simulink model "pm_motor"  (R2022b)
settings: Solver=VariableStepAuto  StartTime=0.0  StopTime=10.0  RelTol=1e-3
values from neighbouring files (symbols this model uses):
  fe = Phif    (= 2.3036)    [pm_params.m]
  J = 0.013    [IM_System_1.m]    (also in IM_System_2.m; IM_System_3.m; IM_System_noPU_4p2p2kw.m; IM_System_noPU_4p2p2kw_1.m)
  Ld = 0.006    [SPM_System_noPU_3p7kw_PI.m]    (also in pm_params.m = 0.8643)
  Lq = 0.0149    [SPM_System_noPU_3p7kw_PI.m]    (also in pm_params.m = 0.8643)
  Rs = 2.5/3    (= 0.833333333333)    [IM_System_1.m]    (also in IM_System_2.m; IM_System_3.m; IM_System_noPU_4p2p2kw.m; IM_System_noPU_4p2p2kw_1.m)
settings Model: Creator=jack  LastModifiedBy=jack

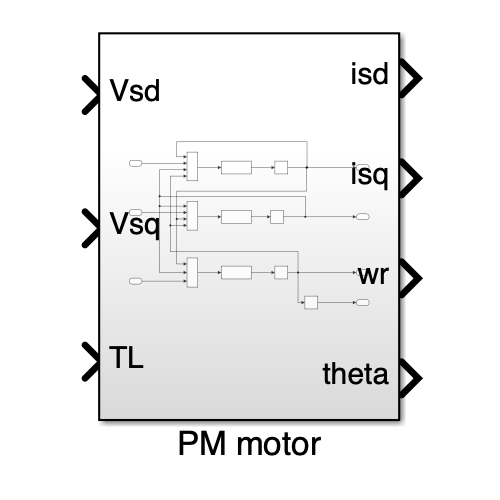
[thumbnail: Simulink's stored preview of the top-level diagram]
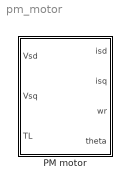
== system pm_motor ==
  PM motor : Subsystem

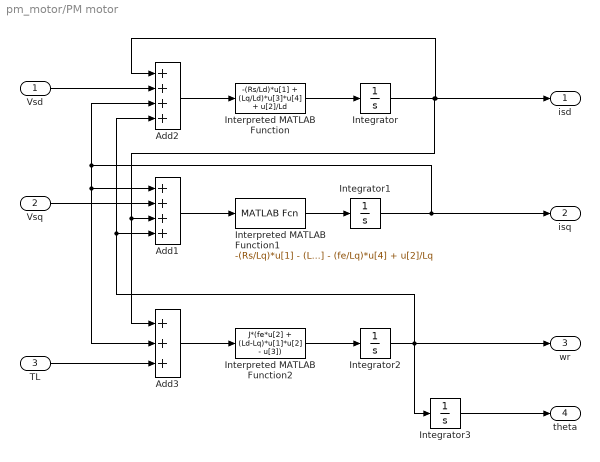
== system pm_motor/PM motor ==
  Vsd : Inport
  Vsq : Inport  Port=2
  TL : Inport  Port=3
  Add1 : Sum  Inputs=++++
  Add2 : Sum  Inputs=++++
  Add3 : Sum  Inputs=+++
  Integrator{,1..3} (4 alike) : Integrator
  Interpreted MATLAB Function : MATLABFcn  MATLABFcn=-(Rs/Ld)*u[1] + (Lq/Ld)*u[3]*u[4] + u[2]/Ld
  Interpreted MATLAB Function1 : MATLABFcn  MATLABFcn=-(Rs/Lq)*u[1] - (Ld/Lq)*u[3]*u[4] - (fe/Lq)*u[4] + u[2]/Lq
  Interpreted MATLAB Function2 : MATLABFcn  MATLABFcn=J*(fe*u[2] + (Ld-Lq)*u[1]*u[2] - u[3])
  isd : Outport
  isq : Outport  Port=2
  wr : Outport  Port=3
  theta : Outport  Port=4
  wires:
  Add1/1 -> Interpreted MATLAB Function1/1
  Integrator3/1 -> theta/1
  Interpreted MATLAB Function/1 -> Integrator/1
  Interpreted MATLAB Function2/1 -> Integrator2/1
  Add3/1 -> Interpreted MATLAB Function2/1
  Integrator/1 -> Add3/1, Add1/3, isd/1, Add2/1
  Add2/1 -> Interpreted MATLAB Function/1
  Integrator1/1 -> isq/1, Add1/1, Add3/2, Add2/3
  Integrator2/1 -> wr/1, Add1/4, Add2/4, Integrator3/1
  Interpreted MATLAB Function1/1 -> Integrator1/1
  TL/1 -> Add3/3
  Vsq/1 -> Add1/2
  Vsd/1 -> Add2/2
